simulink model "iter_impedance"  (R2017b)
settings: Solver=VariableStepAuto  StartTime=0.0  StopTime=3  RelTol=1e-3
libraries: simulink x1
settings Model: Creator=Administrator  LastModifiedBy=Administrator

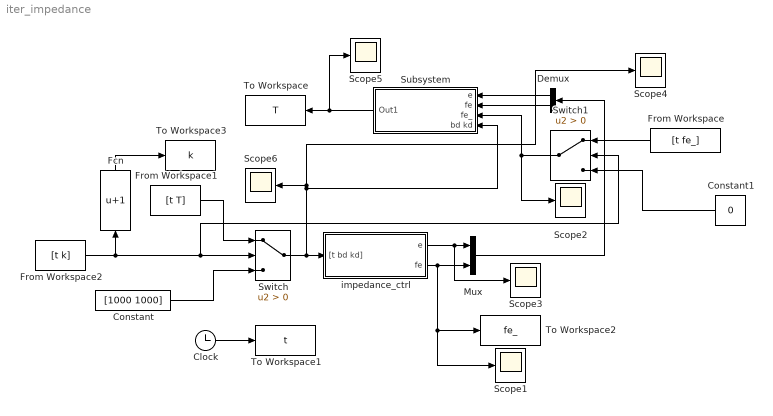
== system iter_impedance ==
  Clock : Clock
  Constant : Constant  Value=[1000 1000]
  Constant1 : Constant  Value=0
  Demux : Demux  Outputs=2
  Fcn : Fcn  Expr=u+1
  From Workspace : FromWorkspace  VariableName=[t fe_]  SampleTime=0
  From Workspace1 : FromWorkspace  VariableName=[t T]  SampleTime=0
  From Workspace2 : FromWorkspace  VariableName=[t k]  SampleTime=0
  Mux : Mux  Inputs=2
  Scope{1..6} (6 alike) : Scope
  Subsystem : Subsystem
  Switch : Switch  Criteria=u2 > Threshold  SaturateOnIntegerOverflow=on
  Switch1 : Switch  Criteria=u2 > Threshold  SaturateOnIntegerOverflow=on
  To Workspace : ToWorkspace  VariableName=T  SampleTime=-1
      settings: Save2DSignal=2-D array (concatenate along first dimension)
  To Workspace1 : ToWorkspace  VariableName=t  SampleTime=0.01
  To Workspace2 : ToWorkspace  VariableName=fe_  SampleTime=0.01
      settings: Save2DSignal=2-D array (concatenate along first dimension)
  To Workspace3 : ToWorkspace  VariableName=k  SampleTime=0.01
  impedance_ctrl : Subsystem
  wires:
  From Workspace1/1 -> Switch/1
  From Workspace2/1 -> Switch1/2, Switch/2, Fcn/1
  Constant/1 -> Switch/3
  Fcn/1 -> To Workspace3/1
  Switch/1 -> Scope6/1, Scope4/1, Subsystem/4(bd kd), impedance_ctrl/1("[t bd kd]")
  impedance_ctrl/1(e) -> Scope3/1, Mux/1
  impedance_ctrl/2(fe) -> Scope1/1, To Workspace2/1, Mux/2
  Mux/1 -> Demux/1
  Demux/1 -> Subsystem/1(e)
  Demux/2 -> Subsystem/2(fe)
  Subsystem/1(Out1) -> Scope5/1, To Workspace/1
  Clock/1 -> To Workspace1/1
  From Workspace/1 -> Switch1/1
  Constant1/1 -> Switch1/3
  Switch1/1 -> Scope2/1, Subsystem/3(fe_)

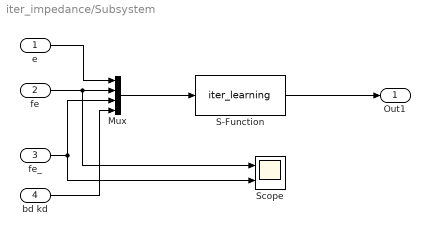
== system iter_impedance/Subsystem ==
  e : Inport
  fe : Inport  Port=2
  fe_ : Inport  Port=3
  bd kd : Inport  Port=4
  Mux : Mux
  S-Function : S-Function  FunctionName=iter_learning  SFunctionDeploymentMode=off  EnableBusSupport=off
  Scope : Scope  NumInputPorts=2
  Out1 : Outport
  wires:
  e/1 -> Mux/1
  fe/1 -> Scope/1, Mux/2
  Mux/1 -> S-Function/1
  bd kd/1 -> Mux/4
  S-Function/1 -> Out1/1
  fe_/1 -> Scope/2, Mux/3

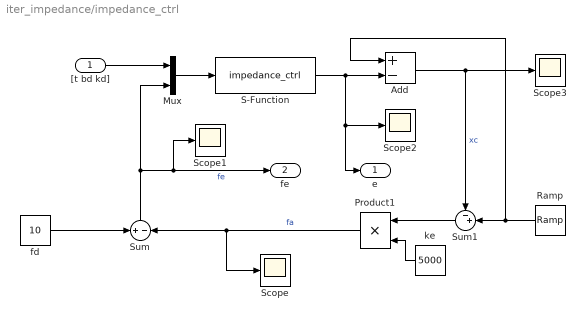
== system iter_impedance/impedance_ctrl ==
  "[t bd kd]" : Inport
  Add : Sum  Inputs=+-
  Mux : Mux  Inputs=2
  Product1 : Product
  Ramp : simulink/Sources/Ramp  slope=1  start=0  X0=0
  S-Function : S-Function  FunctionName=impedance_ctrl  SFunctionDeploymentMode=off  EnableBusSupport=off
  Scope{,1..3} (4 alike) : Scope
  Sum : Sum  Inputs=+|-
  Sum1 : Sum  Inputs=-+|
  fd : Constant  Value=10
  ke : Constant  Value=5000
  e : Outport
  fe : Outport  Port=2
  wires:
  fd/1 -> Sum/1
  Product1/1 -> Scope/1, Sum/2  "fa"
  ke/1 -> Product1/2
  Sum1/1 -> Product1/1
  Add/1 -> Sum1/1, Scope3/1  "xc"
  S-Function/1 -> Scope2/1, e/1, Add/2
  "[t bd kd]"/1 -> Mux/1
  Sum/1 -> Mux/2, Scope1/1, fe/1  "fe"
  Mux/1 -> S-Function/1
  Ramp/1 -> Sum1/2, Add/1
